simulink model "LQR_Example1"  (R2014a)
settings: Solver=ode45  StartTime=0.0  StopTime=10.0  RelTol=1e-3
undefined symbols (not defined in the file): A, B, K
settings Model: Creator=IVDL  LastModifiedBy=user
settings OptimizationCC: SimCompilerOptimization=off
settings DebuggingCC: UnderspecifiedInitializationDetection=Classic  FrameProcessingCompatibilityMsg=error  StateNameClashWarn=warning
settings RTWCC: RTWCompilerOptimization=off
settings ConfigComp: CovMetricSettings=dw  CovHtmlReporting=on  CovSaveCumulativeToWorkspaceVar=on  CovSaveSingleToWorkspaceVar=on  CovModelRefEnable=Off  CovExternalEMLEnable=off

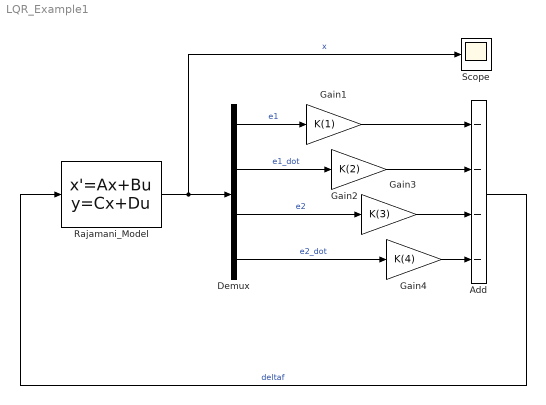
== system LQR_Example1 ==
  Add : Sum  Inputs=----
  Demux : Demux
  Gain1 : Gain  Gain=K(1)
  Gain2 : Gain  Gain=K(2)
  Gain3 : Gain  Gain=K(3)
  Gain4 : Gain  Gain=K(4)
  Rajamani_Model : StateSpace  A=A  B=B  C=eye(4,4)  D=[0;0;0;0]  X0=[3.6/2 0 10*pi/180 0]  ContinuousStateAttributes={'e1','e1_dot','e2','e2_dot'}
  Scope : Scope
  wires:
  Rajamani_Model/1 -> Scope/1, Demux/1  "x"
  Gain4/1 -> Add/4
  Gain3/1 -> Add/3
  Gain2/1 -> Add/2
  Gain1/1 -> Add/1
  Add/1 -> Rajamani_Model/1  "deltaf"
  Demux/1 -> Gain1/1  "e1"
  Demux/2 -> Gain2/1  "e1_dot"
  Demux/3 -> Gain3/1  "e2"
  Demux/4 -> Gain4/1  "e2_dot"
